simulink model "closedLoop_ProductionTest"  (R2019b)
settings: Solver=VariableStepAuto  StartTime=0.0  StopTime=30  RelTol=1e-3
values from neighbouring files (symbols this model uses):
  A_obs = A - L*C    [testClosedLoop_Design.m]    (also in testClosedLoop_Production.m)
  B_obs = [L B - (L*D)]    [testClosedLoop_Design.m]    (also in testClosedLoop_Production.m)
  C_obs = eye(size(A_obs))    [testClosedLoop_Design.m]    (also in testClosedLoop_Production.m)
  D_obs = zeros(size(B_obs))    [testClosedLoop_Design.m]    (also in testClosedLoop_Production.m)
  xhat_init = zeros(n,1)    [testClosedLoop_Design.m]    (also in testClosedLoop_Production.m)
undefined symbols (not defined in the file or in its folder): K
settings Model: Creator=trest  LastModifiedBy=trest

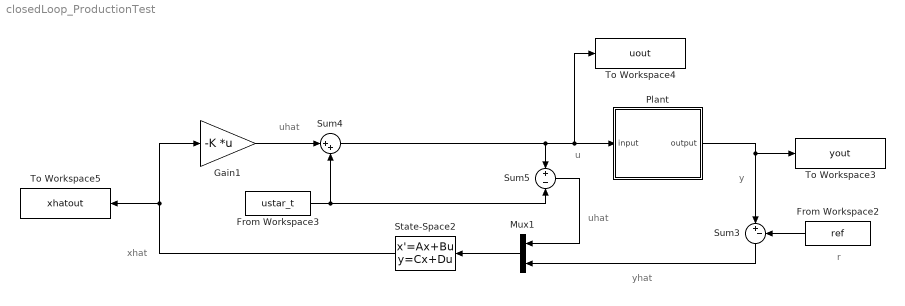
== system closedLoop_ProductionTest ==
  note: uhat
  note: yhat
  note: y
  note: u
  note: xhat
  note: r
  note: uhat
  From Workspace2 : FromWorkspace  VariableName=ref  SampleTime=0
  From Workspace3 : FromWorkspace  VariableName=ustar_t  SampleTime=0
  Gain1 : Gain  Gain=-K  Multiplication=Matrix(K*u)
  Mux1 : Mux  Inputs=2
  Plant : Subsystem
  State-Space2 : StateSpace  A=A_obs  B=B_obs  C=C_obs  D=D_obs  InitialCondition=xhat_init  ContinuousStateAttributes='observer_state'
  Sum3 : Sum  Inputs=|+-
  Sum4 : Sum  Inputs=|++
  Sum5 : Sum  Inputs=+-
  To Workspace3 : ToWorkspace  VariableName=yout  SaveFormat=Timeseries  SampleTime=-1
  To Workspace4 : ToWorkspace  VariableName=uout  SaveFormat=Timeseries  SampleTime=-1
  To Workspace5 : ToWorkspace  VariableName=xhatout  SaveFormat=Timeseries  SampleTime=-1
  wires:
  Sum3/1 -> Mux1/2
  State-Space2/1 -> To Workspace5/1, Gain1/1
  From Workspace2/1 -> Sum3/2
  Gain1/1 -> Sum4/1
  From Workspace3/1 -> Sum4/2, Sum5/2
  Mux1/1 -> State-Space2/1
  Sum5/1 -> Mux1/1
  Plant/1(output) -> To Workspace3/1, Sum3/1
  Sum4/1 -> Plant/1(input), To Workspace4/1, Sum5/1

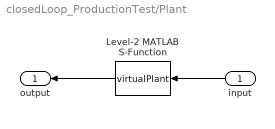
== system closedLoop_ProductionTest/Plant ==
  input : Inport
  Level-2 MATLAB S-Function : M-S-Function  FunctionName=virtualPlant
  output : Outport
  wires:
  input/1 -> Level-2 MATLAB S-Function/1
  Level-2 MATLAB S-Function/1 -> output/1
